simulink model "integracionExperimenta"  (R2023b)
settings: Solver=FixedStepAuto  StartTime=0.0  StopTime=2.0  RelTol=1e-3  EnableMultiTasking=on
settings Model: ExtModeTrigDuration=2  Creator=fdcdm  LastModifiedBy=Carlos
settings OptimizationCC: EnhancedBackFolding=on  PassReuseOutputArgsAs=Individual arguments  ZeroExternalMemoryAtStartup=off  ZeroInternalMemoryAtStartup=off  MaxStackSize=64  OptimizeBlockOrder=speed  DifferentSizesBufferReuse=on  OptimizationCustomize=off  EfficientTunableParamExpr=on
settings DebuggingCC: ParameterTunabilityLossMsg=error
settings HardwareCC: ProdBitPerInt=16  ProdBitPerPointer=16  ProdBitPerSizeT=16  ProdBitPerPtrDiffT=16  ProdLargestAtomicFloat=None  ProdWordSize=8  ProdHWDeviceType=Atmel->AVR  UseEmbeddedCoderFeatures=off  UseSimulinkCoderFeatures=off
settings SFSimCC: MATLABDynamicMemAlloc=off
settings RTWCC: Description=Embedded Coder  SystemTargetFile=ert.tlc  HardwareBoard=Arduino Mega 2560  TemplateMakefile=ert_default_tmf  Toolchain=Arduino AVR  BuildConfiguration=Faster Runs
settings CodeAppCC: ForceParamTrailComments=on  IgnoreCustomStorageClasses=off  OperatorAnnotations=on  SimulinkDataObjDesc=on  SFDataObjDesc=on  InsertBlockDesc=on
settings ERTTargetCC: SupportContinuousTime=on  SupportNonInlinedSFcns=on  SupportVariableSizeSignals=on  ExtModeTransport=3  ExtModeStaticAlloc=on  ExtModeAutomaticAllocSize=off  ExtModeStaticAllocSize=2048  ExtModeMexFile=ext_xcp  ExtModeIntrfLevel=Level2 - Open

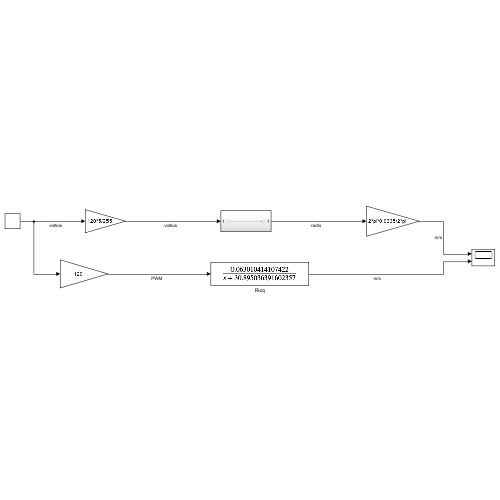
[thumbnail: Simulink's stored preview of the top-level diagram]
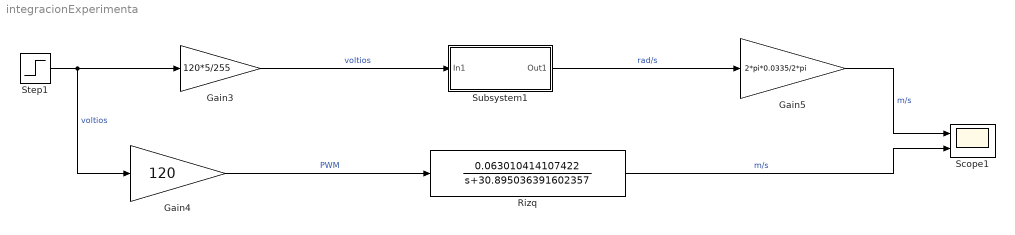
== system integracionExperimenta ==
  Gain3 : Gain  Gain=120*5/255
  Gain4 : Gain  Gain=120
  Gain5 : Gain  Gain=2*pi*0.0335/2*pi
  Rizq : TransferFcn  Numerator=0.063010414107422  Denominator=[1,30.895036391602357]
  Scope1 : Scope  NumInputPorts=2
  Step1 : Step  SampleTime=0
  Subsystem1 : Subsystem
  wires:
  Subsystem1/1(Out1) -> Gain5/1  "rad/s"
  Gain5/1 -> Scope1/1  "m/s"
  Step1/1 -> Gain4/1, Gain3/1  "voltios"
  Gain3/1 -> Subsystem1/1(In1)  "voltios"
  Rizq/1 -> Scope1/2  "m/s"
  Gain4/1 -> Rizq/1  "PWM"

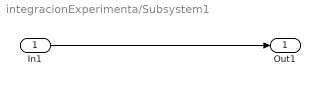
== system integracionExperimenta/Subsystem1 ==
  In1 : Inport
  Out1 : Outport
  wires:
  In1/1 -> Out1/1
